simulink model "mo2_1"  (R2024b)
settings: Solver=VariableStepAuto  StartTime=0.0  StopTime=10.0  RelTol=1e-3
settings Model: Creator=24839  LastModifiedBy=24839

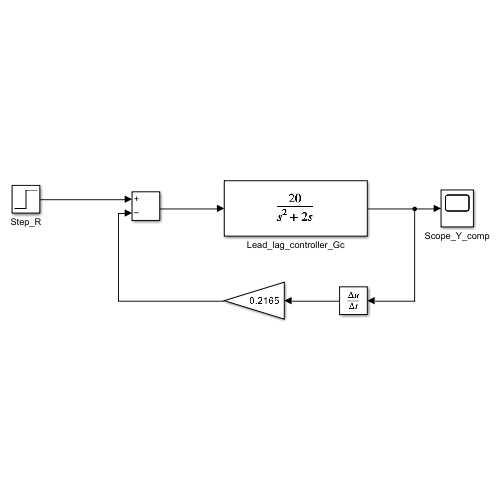
[thumbnail: Simulink's stored preview of the top-level diagram]
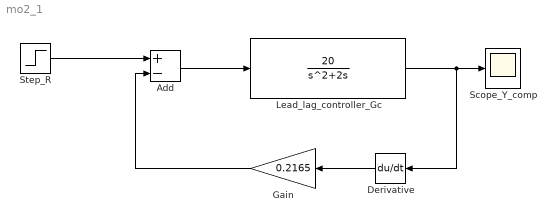
== system mo2_1 ==
  Add : Sum  Inputs=+-
  Derivative : Derivative
  Gain : Gain  Gain=0.2165
  Lead_lag_controller_Gc : TransferFcn  Numerator=20  Denominator=[1 2 0]
  Scope_Y_comp : Scope
  Step_R : Step  Time=0  SampleTime=0
  wires:
  Lead_lag_controller_Gc/1 -> Derivative/1, Scope_Y_comp/1
  Add/1 -> Lead_lag_controller_Gc/1
  Derivative/1 -> Gain/1
  Gain/1 -> Add/2
  Step_R/1 -> Add/1
